simulink model "AltBaroInertial"  (R2023a)
settings: Solver=ode5  StartTime=0.0  StopTime=10.0  FixedStep=0.1  RelTol=1e-3
undefined symbols (not defined in the file or in its folder): Ah, Al, Bh, Bl
libraries: simulink x2
settings Model: Creator=dany0  LastModifiedBy=Utente
settings DataIOCC: SaveFormat=Array

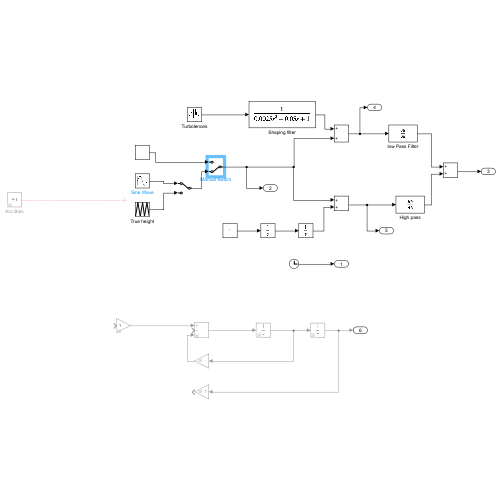
[thumbnail: Simulink's stored preview of the top-level diagram]
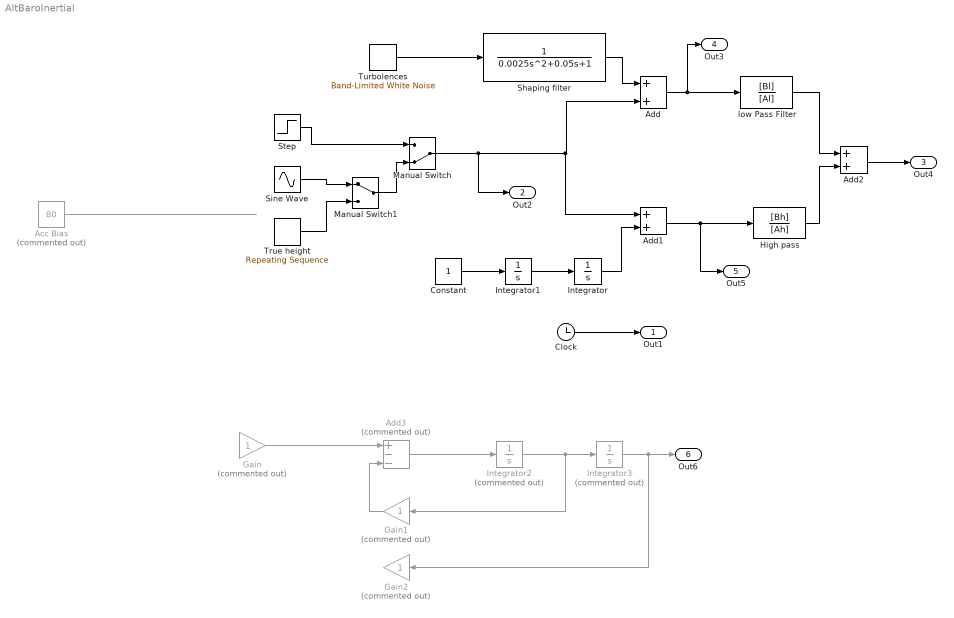
== system AltBaroInertial ==
  Acc Bias : Constant  Commented=on  Value=80
  Add : Sum
  Add1 : Sum
  Add2 : Sum
  Add3 : Sum  Commented=on  Inputs=+--
  Clock : Clock
  Constant : Constant
  Gain : Gain  Commented=on
  Gain1 : Gain  Commented=on
  Gain2 : Gain  Commented=on
  High pass : TransferFcn  Numerator=[Bh]  Denominator=[Ah]
  Integrator : Integrator
  Integrator1 : Integrator
  Integrator2 : Integrator  Commented=on
  Integrator3 : Integrator  Commented=on
  Manual Switch : ManualSwitch  CurrentSetting=0
  Manual Switch1 : ManualSwitch
  Shaping filter : TransferFcn  Denominator=[0.0025 0.05 1]
  Sine Wave : Sin  Amplitude=100  SampleTime=0
  Step : Step  Time=5  After=100  SampleTime=0
  True height : simulink/Sources/Repeating Sequence  rep_seq_t=[0 10 20]  rep_seq_y=[100 200 100]
  Turbolences : simulink/Sources/Band-Limited White Noise  Cov=[5]  Ts=0.1  seed=[23341]
  low Pass Filter : TransferFcn  Numerator=[Bl]  Denominator=[Al]
  Out1 : Outport
  Out2 : Outport  Port=2
  Out4 : Outport  Port=3
  Out3 : Outport  Port=4
  Out5 : Outport  Port=5
  Out6 : Outport  Port=6
  wires:
  Turbolences/1 -> Shaping filter/1
  Shaping filter/1 -> Add/1
  Add/1 -> Out3/1, low Pass Filter/1
  Add1/1 -> Out5/1, High pass/1
  High pass/1 -> Add2/2
  low Pass Filter/1 -> Add2/1
  Add2/1 -> Out4/1
  Clock/1 -> Out1/1
  Add3/1 -> Integrator2/1
  Integrator2/1 -> Gain1/1, Integrator3/1
  Integrator3/1 -> Gain2/1, Out6/1
  Gain/1 -> Add3/1
  Gain1/1 -> Add3/3
  Constant/1 -> Integrator1/1
  Integrator1/1 -> Integrator/1
  Integrator/1 -> Add1/2
  Acc Bias/1 -> ?
  Manual Switch/1 -> Out2/1, Add1/1, Add/2
  Step/1 -> Manual Switch/1
  Sine Wave/1 -> Manual Switch1/1
  True height/1 -> Manual Switch1/2
  Manual Switch1/1 -> Manual Switch/2
